simulink model "Lab2Simulink"  (R2023a)
settings: Solver=VariableStepAuto  StartTime=0.0  StopTime=20.0  RelTol=1e-3
settings Model: Creator=santi  LastModifiedBy=santi

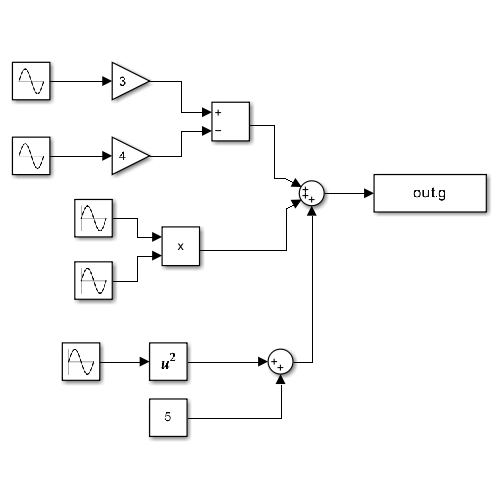
[thumbnail: Simulink's stored preview of the top-level diagram]
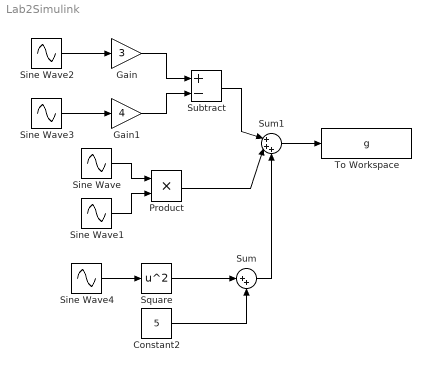
== system Lab2Simulink ==
  Constant2 : Constant  Value=5
  Gain : Gain  Gain=3
  Gain1 : Gain  Gain=4
  Product : Product
  Sine Wave : Sin  Frequency=6.28  SampleTime=0
  Sine Wave1 : Sin  Amplitude=2  Frequency=0.63  Phase=90  SampleTime=0
  Sine Wave2 : Sin  Frequency=6.28  SampleTime=0
  Sine Wave3 : Sin  Amplitude=2  Frequency=0.63  Phase=90  SampleTime=0
  Sine Wave4 : Sin  Frequency=6.28  SampleTime=0
  Square : Math  Operator=square
  Subtract : Sum  Inputs=+-
  Sum : Sum  Inputs=|++
  Sum1 : Sum  Inputs=|+++
  To Workspace : ToWorkspace  VariableName=g  SaveFormat=Structure With Time  SampleTime=-1
  wires:
  Sine Wave/1 -> Product/1
  Sine Wave2/1 -> Gain/1
  Sine Wave4/1 -> Square/1
  Square/1 -> Sum/1
  Constant2/1 -> Sum/2
  Subtract/1 -> Sum1/1
  Product/1 -> Sum1/2
  Sum/1 -> Sum1/3
  Gain/1 -> Subtract/1
  Sine Wave3/1 -> Gain1/1
  Gain1/1 -> Subtract/2
  Sine Wave1/1 -> Product/2
  Sum1/1 -> To Workspace/1
